simulink model "Ex2_2_sim"  (R2017b)
settings: Solver=ode45  StartTime=0.0  StopTime=Endtime  RelTol=1e-3
settings Model: Creator=Shin  LastModifiedBy=minakata
settings DataIOCC: LimitDataPoints=on  SaveFormat=Array
settings OptimizationCC: BlockReduction=off  BooleanDataType=off  LifeSpan=inf
settings DebuggingCC: SaveWithParameterizedLinksMsg=none  UnderspecifiedInitializationDetection=Classic  MergeDetectMultiDrivingBlocksExec=none  SignalResolutionControl=TryResolveAllWithWarning  SFUnexpectedBacktrackingDiag=warning  SFNoUnconditionalDefaultTransitionDiag=warning  SFExecutionAtInitializationDiag=none
settings HardwareCC: ProdBitPerPointer=32  ProdBitPerSizeT=32  ProdBitPerPtrDiffT=32  ProdLargestAtomicFloat=None  ProdIntDivRoundTo=Undefined  ProdEndianess=Unspecified  ProdWordSize=32  ProdHWDeviceType=32-bit Generic  TargetUnknown=on
settings ModelReferenceCC: PropagateSignalLabelsOutOfModel=off
settings CodeAppCC: StateflowObjectComments=on
settings GRTTargetCC: TargetLangStandard=C89/C90 (ANSI)  GeneratePreprocessorConditionals=Disable all
settings ConfigComp: CovMetricSettings=dw  CovHtmlReporting=on  CovSaveCumulativeToWorkspaceVar=on  CovSaveSingleToWorkspaceVar=on  CovExternalEMLEnable=off

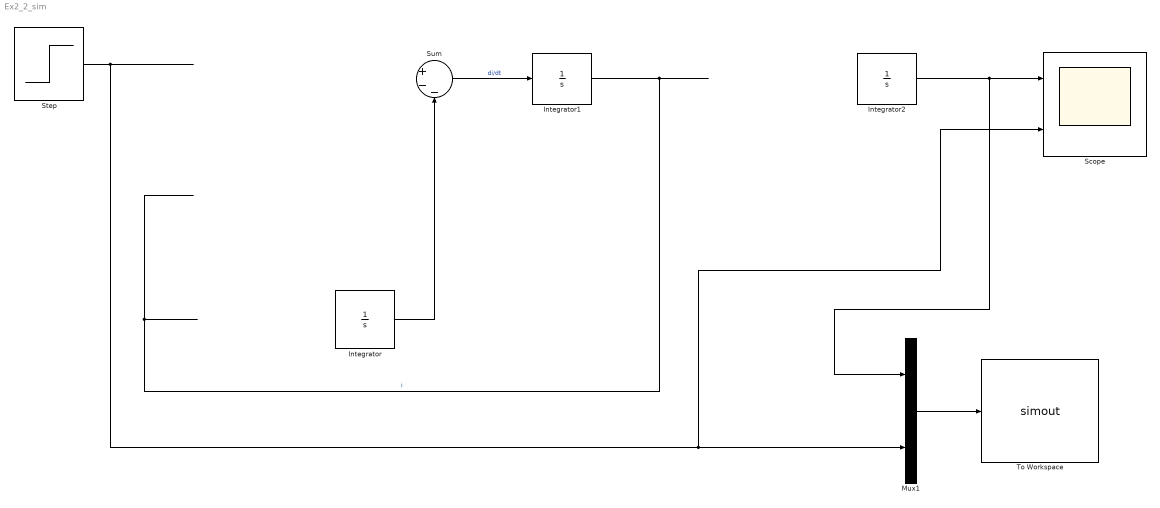
== system Ex2_2_sim ==
  Integrator : Integrator
  Integrator1 : Integrator
  Integrator2 : Integrator
  Mux1 : Mux  Inputs=2
  Scope : Scope  NumInputPorts=2
  Step : Step  Time=1e-4  SampleTime=0
  Sum : Sum  Inputs=|+--
  To Workspace : ToWorkspace  VariableName=simout  SaveFormat=Timeseries  SampleTime=-1
  wires:
  Step/1 -> Scope/2, Mux1/2
  ? -> Sum/1
  ? -> Sum/2
  Sum/1 -> Integrator1/1  "di/dt"
  ? -> Integrator/1
  Integrator/1 -> Sum/3
  Integrator1/1 -> ?  "i"
  ? -> Integrator2/1
  Integrator2/1 -> Mux1/1, Scope/1
  Mux1/1 -> To Workspace/1
